simulink model "Copy_of_modelo_completo"  (R2021a)
settings: Solver=VariableStepAuto  StartTime=0.0  StopTime=10.0  RelTol=1e-3
values from neighbouring files (symbols this model uses):
  bah = Meqh*nh*w_posh    (= 720000)    [Data.m]
  bat = Meqt*nt*w_post    (= 675000)    [Data.m]
  bcx = 1000.0    (= 1000)    [Data.m]
  bcy = 500.0    (= 500)    [Data.m]
  beqh = 18.0    (= 18)    [Data.m]
  beqhd = bh + ((beqh*(rth^2))/(Rd^2))    (= 28800)    [Data.m]
  beqt = bt + (beq_rot*rt^2)/(Rw^2)    (= 27000)    [Data.m]
  bw = 30000.0    (= 30000)    [Data.m]
  cont_mass = max_m    (= 50000)    [Data.m]
  ddxmax = 1    [Data.m]
  ddxmin = -1    [Data.m]
  g = 9.80665    [Data.m]    (also in PD_balanceo.m = 9.81)
  Kcy = 1.3e6    (= 1300000)    [Data.m]
  Ksah = Meqh*nh*w_posh^2    (= 4318720.37915)    [Data.m]
  Ksat = Meqt*nt*w_post^2    (= 3088564.26247)    [Data.m]
  Ksiah = Meqh*w_posh^3    (= 10361858.7296)    [Data.m]
  Ksiat = Meqt*w_post^3    (= 5652876.56499)    [Data.m]
  Kw = 1800000.0    (= 1800000)    [Data.m]
  Meqh = Mh + (Jmh*rth^2 + Jd)/Rd^2    (= 48014.2222222)    [Data.m]
  Meqt = mt + (Jw+Jm*rt^2)/(Rw^2)    (= 59008)    [Data.m]
  Rd = 0.75    [Data.m]
  rt = 15.0    (= 15)    [Data.m]    (also in main.m = 0)
  rth = 30.0    (= 30)    [Data.m]
  Rw = 0.5    [Data.m]    (also in main.m = 0)
  sp_mass = 15000.0    (= 15000)    [Data.m]
  yt0 = 45.0    (= 45)    [Data.m]
settings Model: Creator=Mariano  LastModifiedBy=facu_

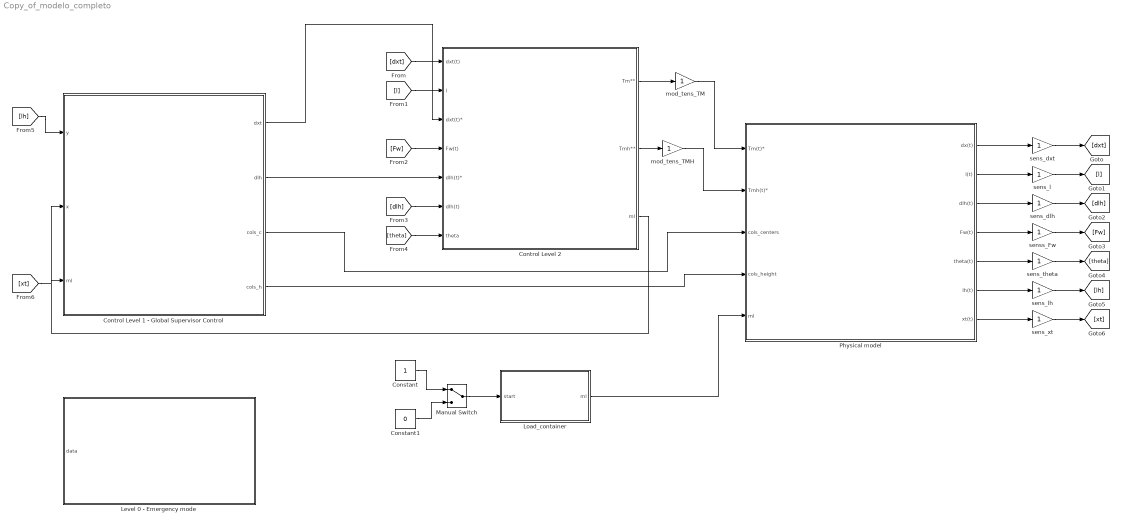
== system Copy_of_modelo_completo ==
  Constant : Constant
  Constant1 : Constant  Value=0
  Control Level 1 - Global Supervisor Control : Stateflow chart  TreatAsAtomicUnit=on
  Control Level 2 : Subsystem
  Level 0 - Emergency mode : Stateflow chart  TreatAsAtomicUnit=on
  Load_container : Subsystem
  Manual Switch : ManualSwitch
  Physical model : Subsystem
  mod_tens_TM : Gain
  mod_tens_TMH : Gain
  sens_dlh : Gain
  sens_dxt : Gain
  sens_l : Gain
  sens_lh : Gain
  sens_theta : Gain
  sens_xt : Gain
  senss_Fw : Gain
  wires:
  Control Level 2/1(Tm**) -> mod_tens_TM/1
  Control Level 2/2(Tmh**) -> mod_tens_TMH/1
  Control Level 1 - Global Supervisor Control/1(dxt) -> Control Level 2/3(dxt(t)*)
  Control Level 1 - Global Supervisor Control/2(dlh) -> Control Level 2/5(dlh(t)*)
  Physical model/1(dx(t)) -> sens_dxt/1
  Physical model/2(l(t)) -> sens_l/1
  Physical model/3(dlh(t)) -> sens_dlh/1
  Physical model/4(Fw(t)) -> senss_Fw/1
  Physical model/5(theta(t)) -> sens_theta/1
  [dxt] -> Control Level 2/1(dxt(t))
  [l] -> Control Level 2/2(l)
  [Fw] -> Control Level 2/4(Fw(t))
  [dlh] -> Control Level 2/6(dlh(t))
  [theta] -> Control Level 2/7(theta)
  Physical model/6(lh(t)) -> sens_lh/1
  Physical model/7(xt(t)) -> sens_xt/1
  [lh] -> Control Level 1 - Global Supervisor Control/1(y)
  [xt] -> Control Level 1 - Global Supervisor Control/2(x)
  sens_dxt/1 -> [dxt]
  sens_l/1 -> [l]
  sens_dlh/1 -> [dlh]
  senss_Fw/1 -> [Fw]
  sens_theta/1 -> [theta]
  sens_lh/1 -> [lh]
  sens_xt/1 -> [xt]
  mod_tens_TM/1 -> Physical model/1(Tm(t)*)
  mod_tens_TMH/1 -> Physical model/2(Tmh(t)*)
  Control Level 1 - Global Supervisor Control/3(cols_c) -> Physical model/3(cols_centers)
  Control Level 1 - Global Supervisor Control/4(cols_h) -> Physical model/4(cols_height)
  Load_container/1(ml) -> Physical model/5(ml)
  Manual Switch/1 -> Load_container/1(start)
  Constant/1 -> Manual Switch/1
  Constant1/1 -> Manual Switch/2
  Control Level 2/3(ml) -> Control Level 1 - Global Supervisor Control/3(ml)

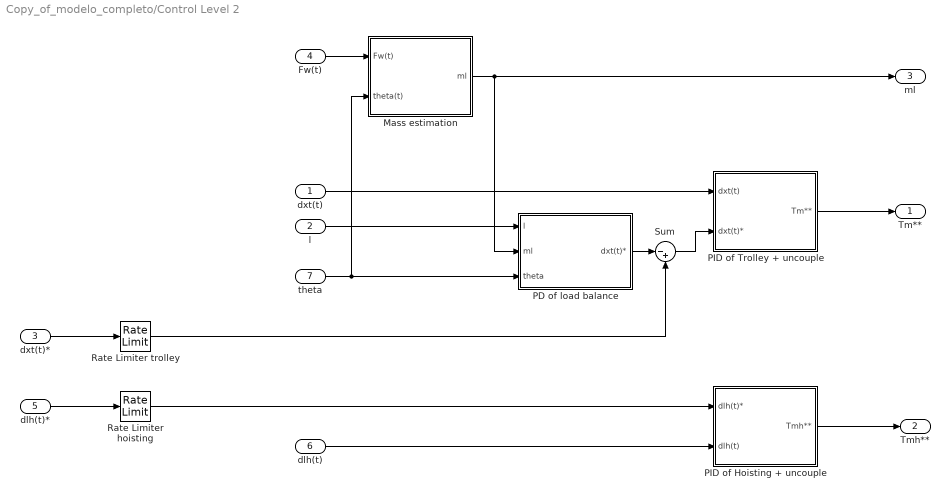
== system Copy_of_modelo_completo/Control Level 2 ==
  dxt(t) : Inport
  l : Inport  Port=2
  dxt(t)* : Inport  Port=3
  Fw(t) : Inport  Port=4
  dlh(t)* : Inport  Port=5
  dlh(t) : Inport  Port=6
  theta : Inport  Port=7
  Mass estimation : Subsystem
  "PD of load balance " : Subsystem
  "PID of Hoisting + uncouple " : Subsystem
  "PID of Trolley + uncouple " : Subsystem
  Rate Limiter hoisting : RateLimiter  RisingSlewLimit=ddxmax  FallingSlewLimit=ddxmin
  Rate Limiter trolley : RateLimiter  RisingSlewLimit=ddxmax  FallingSlewLimit=ddxmin
  Sum : Sum  Inputs=|-+
  Tm** : Outport
  Tmh** : Outport  Port=2
  ml : Outport  Port=3
  wires:
  dlh(t)*/1 -> Rate Limiter hoisting/1
  Fw(t)/1 -> Mass estimation/1(Fw(t))
  "PID of Trolley + uncouple "/1(Tm**) -> Tm**/1
  Mass estimation/1(ml) -> ml/1, "PD of load balance "/2(ml)
  "PD of load balance "/1(dxt(t)*) -> Sum/1
  Sum/1 -> "PID of Trolley + uncouple "/2(dxt(t)*)
  dxt(t)/1 -> "PID of Trolley + uncouple "/1(dxt(t))
  "PID of Hoisting + uncouple "/1(Tmh**) -> Tmh**/1
  dxt(t)*/1 -> Rate Limiter trolley/1
  l/1 -> "PD of load balance "/1(l)
  theta/1 -> Mass estimation/2(theta(t)), "PD of load balance "/3(theta)
  Rate Limiter trolley/1 -> Sum/2
  Rate Limiter hoisting/1 -> "PID of Hoisting + uncouple "/1(dlh(t)*)
  dlh(t)/1 -> "PID of Hoisting + uncouple "/2(dlh(t))

== system Copy_of_modelo_completo/Load_container ==
  start : Inport
  Sum : Sum  Inputs=|++
  Switch : Switch  Criteria=u2 > Threshold
  no_container : Constant  Value=0
  random_container_mass : Constant  Value=cont_mass
  spreader mass : Constant  Value=sp_mass
  ml : Outport
  wires:
  no_container/1 -> Switch/1
  spreader mass/1 -> Sum/2
  random_container_mass/1 -> Switch/3
  Switch/1 -> Sum/1
  Sum/1 -> ml/1
  start/1 -> Switch/2

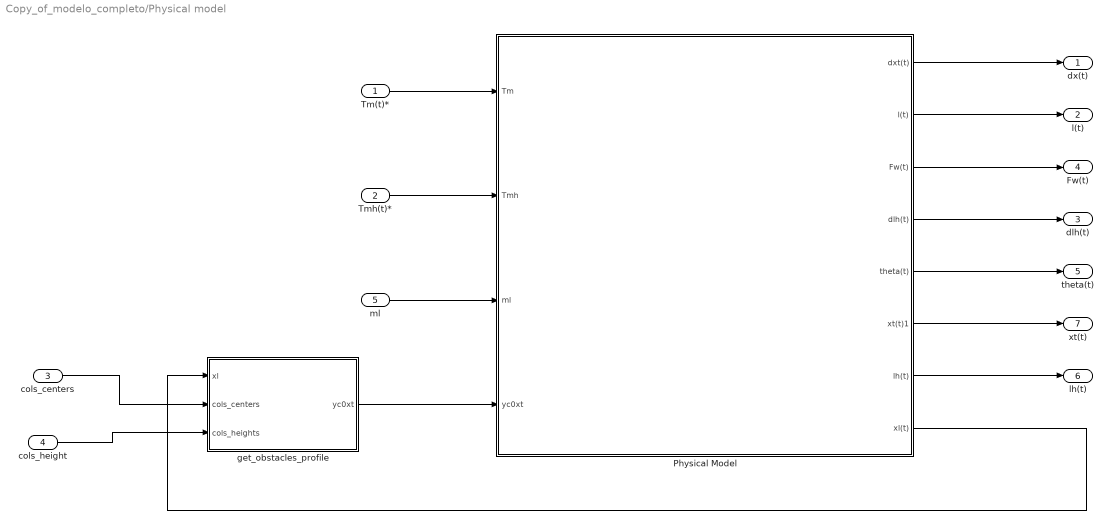
== system Copy_of_modelo_completo/Physical model ==
  Tm(t)* : Inport
  Tmh(t)* : Inport  Port=2
  cols_centers : Inport  Port=3
  cols_height : Inport  Port=4
  ml : Inport  Port=5
  Physical Model : Subsystem
  get_obstacles_profile : MATLAB Function  TreatAsAtomicUnit=on
  dx(t) : Outport
  l(t) : Outport  Port=2
  dlh(t) : Outport  Port=3
  Fw(t) : Outport  Port=4
  theta(t) : Outport  Port=5
  lh(t) : Outport  Port=6
  xt(t) : Outport  Port=7
  wires:
  Physical Model/4(dlh(t)) -> dlh(t)/1
  Physical Model/2(l(t)) -> l(t)/1
  Physical Model/1(dxt(t)) -> dx(t)/1
  Physical Model/3(Fw(t)) -> Fw(t)/1
  Physical Model/5(theta(t)) -> theta(t)/1
  Physical Model/6(xt(t)1) -> xt(t)/1
  Physical Model/7(lh(t)) -> lh(t)/1
  Tmh(t)*/1 -> Physical Model/2(Tmh)
  Tm(t)*/1 -> Physical Model/1(Tm)
  ml/1 -> Physical Model/3(ml)
  get_obstacles_profile/1(yc0xt) -> Physical Model/4(yc0xt)
  Physical Model/8(xl(t)) -> get_obstacles_profile/1(xl)
  cols_centers/1 -> get_obstacles_profile/2(cols_centers)
  cols_height/1 -> get_obstacles_profile/3(cols_heights)

== system Copy_of_modelo_completo/Control Level 2/Mass estimation ==
  Fw(t) : Inport
  theta(t) : Inport  Port=2
  Constant : Constant  Value=g
  Divide : Product  Inputs=*/
  Product : Product
  Trigonometric Function : Trigonometry
  ml : Outport
  wires:
  theta(t)/1 -> Trigonometric Function/1
  Trigonometric Function/1 -> Product/2
  Fw(t)/1 -> Product/1
  Divide/1 -> ml/1
  Product/1 -> Divide/1
  Constant/1 -> Divide/2

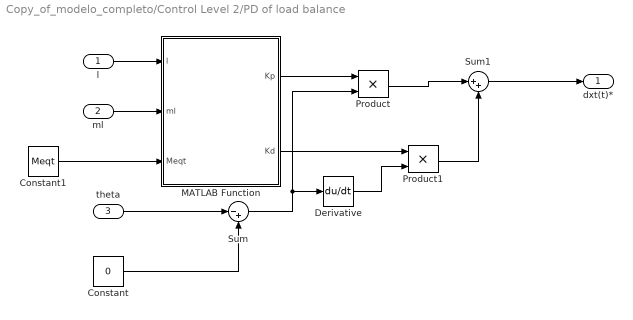
== system Copy_of_modelo_completo/Control Level 2/PD of load balance  ==
  l : Inport
  ml : Inport  Port=2
  theta : Inport  Port=3
  Constant : Constant  Value=0
  Constant1 : Constant  Value=Meqt
  Derivative : Derivative
  MATLAB Function : MATLAB Function  TreatAsAtomicUnit=on
  Product : Product
  Product1 : Product
  Sum : Sum  Inputs=|-+
  Sum1 : Sum  Inputs=|++
  dxt(t)* : Outport
  wires:
  theta/1 -> Sum/1
  Constant/1 -> Sum/2
  ml/1 -> MATLAB Function/2(ml)
  Sum/1 -> Product/2, Derivative/1
  Product1/1 -> Sum1/2
  Product/1 -> Sum1/1
  Sum1/1 -> dxt(t)*/1
  MATLAB Function/2(Kd) -> Product1/1
  MATLAB Function/1(Kp) -> Product/1
  Derivative/1 -> Product1/2
  l/1 -> MATLAB Function/1(l)
  Constant1/1 -> MATLAB Function/3(Meqt)

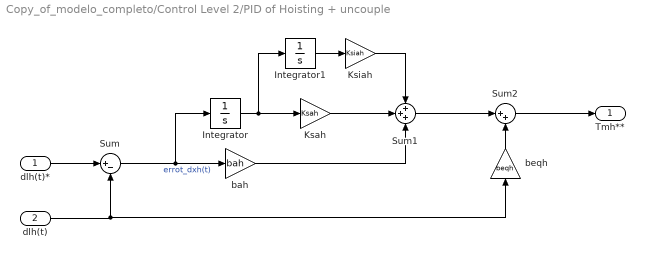
== system Copy_of_modelo_completo/Control Level 2/PID of Hoisting + uncouple  ==
  dlh(t)* : Inport
  dlh(t) : Inport  Port=2
  Integrator : Integrator
  Integrator1 : Integrator
  Ksah : Gain  Gain=Ksah
  Ksiah : Gain  Gain=Ksiah
  Sum : Sum  Inputs=|+-
  Sum1 : Sum  Inputs=+++
  Sum2 : Sum  Inputs=|++
  bah : Gain  Gain=bah
  beqh : Gain  Gain=beqh
  Tmh** : Outport
  wires:
  Sum/1 -> bah/1, Integrator/1  "errot_dxh(t)"
  dlh(t)*/1 -> Sum/1
  Sum1/1 -> Sum2/1
  dlh(t)/1 -> beqh/1, Sum/2
  Integrator/1 -> Integrator1/1, Ksah/1
  bah/1 -> Sum1/3
  Ksah/1 -> Sum1/2
  Integrator1/1 -> Ksiah/1
  Ksiah/1 -> Sum1/1
  beqh/1 -> Sum2/2
  Sum2/1 -> Tmh**/1

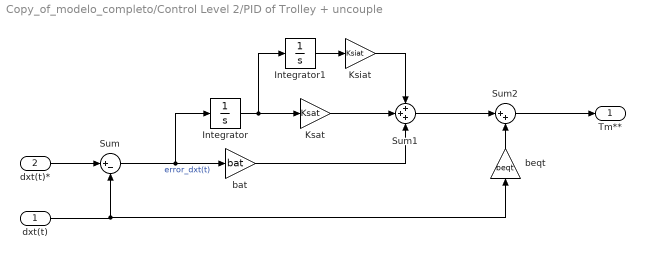
== system Copy_of_modelo_completo/Control Level 2/PID of Trolley + uncouple  ==
  dxt(t) : Inport
  dxt(t)* : Inport  Port=2
  Integrator : Integrator
  Integrator1 : Integrator
  Ksat : Gain  Gain=Ksat
  Ksiat : Gain  Gain=Ksiat
  Sum : Sum  Inputs=|+-
  Sum1 : Sum  Inputs=+++
  Sum2 : Sum  Inputs=|++
  bat : Gain  Gain=bat
  beqt : Gain  Gain=beqt
  Tm** : Outport
  wires:
  Sum/1 -> bat/1, Integrator/1  "error_dxt(t)"
  dxt(t)*/1 -> Sum/1
  Sum1/1 -> Sum2/1
  dxt(t)/1 -> beqt/1, Sum/2
  Integrator/1 -> Integrator1/1, Ksat/1
  bat/1 -> Sum1/3
  Ksat/1 -> Sum1/2
  Integrator1/1 -> Ksiat/1
  Ksiat/1 -> Sum1/1
  beqt/1 -> Sum2/2
  Sum2/1 -> Tm**/1

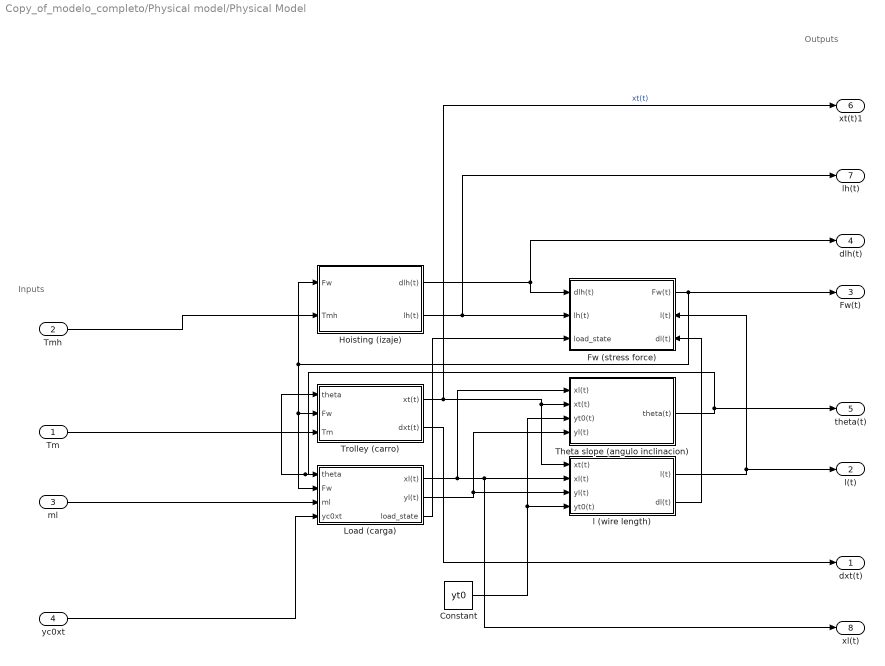
== system Copy_of_modelo_completo/Physical model/Physical Model ==
  note: Inputs
  note: Outputs
  Tm : Inport
  Tmh : Inport  Port=2
  ml : Inport  Port=3
  yc0xt : Inport  Port=4
  Constant : Constant  Value=yt0
  Fw (stress force) : Subsystem
      settings: PortSchema="{\"entries\":[{\"content\":{\"sides\":[{\"content\":{\"connectorIds\":[\"In1\",\"In2\",\"In3\"]},\"type\":\"ConnectorPlacement.EquallySpacedRectSide\",\"uuid\":\"ba23d8a5-df88-4a98-9228-1a95ef0572d6\"},{\"content\":{\"connectorIds\":[\"Out1\",\"In4\",\"In5\"],\"side\":\"RIGHT\"},\"type\":\"ConnectorPlacement.EquallySpacedRectSide\",\"uuid\":\"c1b2cc2a-1d19-40da-89ec-405abbf25b58\"},{\"content\":{\"connectorIds\":[],\"side\":\"TOP\"},\"type\":\"ConnectorPlacement.EquallySpacedRectSide\",\"uuid\":\"8c283652-7118-429a-8320-3bc0966db205\"}]},\"type\":\"ConnectorPlacement.EquallySpacedConnector\",\"uuid\":\"7ebc4a5f-6f80-4333-9ee6-9a21b2f2a5d0\"}],\"packageUris\":[\"http://schema.mathworks.com/mf0/Connector/R2020b\"],\"version\":\"1.0\"}"
  Hoisting (izaje) : Subsystem
  Load (carga) : Subsystem
  Theta slope (angulo inclinacion) : Subsystem
  Trolley (carro) : Subsystem
  l (wire length) : Subsystem
  dxt(t) : Outport
  l(t) : Outport  Port=2
  Fw(t) : Outport  Port=3
  dlh(t) : Outport  Port=4
  theta(t) : Outport  Port=5
  xt(t)1 : Outport  Port=6
  lh(t) : Outport  Port=7
  xl(t) : Outport  Port=8
  wires:
  Theta slope (angulo inclinacion)/1(theta(t)) -> theta(t)/1, Trolley (carro)/1(theta), Load (carga)/1(theta)
  Load (carga)/1(xl(t)) -> xl(t)/1, l (wire length)/2(xl(t)), Theta slope (angulo inclinacion)/1(xl(t))
  Hoisting (izaje)/2(lh(t)) -> lh(t)/1, Fw (stress force)/2(lh(t))
  Trolley (carro)/1(xt(t)) -> xt(t)1/1, l (wire length)/1(xt(t)), Theta slope (angulo inclinacion)/2(xt(t))  "xt(t)"
  Fw (stress force)/1(Fw(t)) -> Trolley (carro)/2(Fw), Load (carga)/2(Fw), Hoisting (izaje)/1(Fw), Fw(t)/1
  Constant/1 -> Theta slope (angulo inclinacion)/3(yt0(t)), l (wire length)/4(yt0(t))
  Load (carga)/2(yl(t)) -> Theta slope (angulo inclinacion)/4(yl(t)), l (wire length)/3(yl(t))
  l (wire length)/1(l(t)) -> l(t)/1, Fw (stress force)/4(l(t))
  ml/1 -> Load (carga)/3(ml)
  l (wire length)/2(dl(t)) -> Fw (stress force)/5(dl(t))
  Tmh/1 -> Hoisting (izaje)/2(Tmh)
  Tm/1 -> Trolley (carro)/3(Tm)
  Hoisting (izaje)/1(dlh(t)) -> Fw (stress force)/1(dlh(t)), dlh(t)/1
  Trolley (carro)/2(dxt(t)) -> dxt(t)/1
  Load (carga)/3(load_state) -> Fw (stress force)/3(load_state)
  yc0xt/1 -> Load (carga)/4(yc0xt)

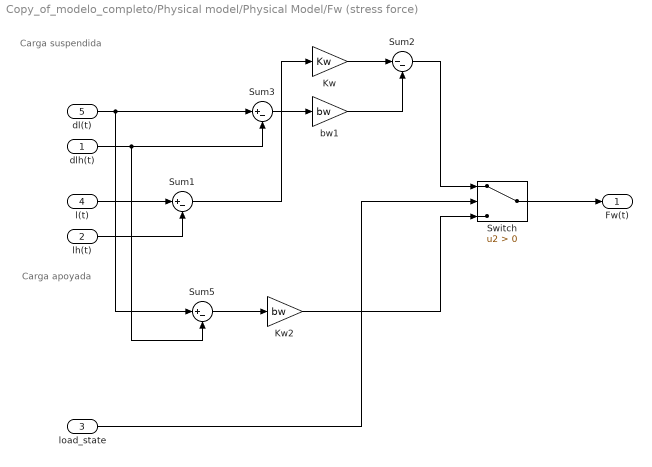
== system Copy_of_modelo_completo/Physical model/Physical Model/Fw (stress force) ==
  note: Carga suspendida
  note: Carga apoyada
  dlh(t) : Inport
  lh(t) : Inport  Port=2
  load_state : Inport  Port=3
  l(t) : Inport  Port=4
  dl(t) : Inport  Port=5
  Kw : Gain  Gain=Kw
  Kw2 : Gain  Gain=bw
  Sum1 : Sum  Inputs=|+-
  Sum2 : Sum  Inputs=|--
  Sum3 : Sum  Inputs=|+-
  Sum5 : Sum  Inputs=|+-
  Switch : Switch  Criteria=u2 > Threshold
  bw1 : Gain  Gain=bw
  Fw(t) : Outport
  wires:
  Switch/1 -> Fw(t)/1
  l(t)/1 -> Sum1/1
  lh(t)/1 -> Sum1/2
  Sum1/1 -> Kw/1
  Sum3/1 -> bw1/1
  bw1/1 -> Sum2/2
  Kw/1 -> Sum2/1
  Sum2/1 -> Switch/1
  Sum5/1 -> Kw2/1
  dlh(t)/1 -> Sum5/2, Sum3/2
  dl(t)/1 -> Sum5/1, Sum3/1
  Kw2/1 -> Switch/3
  load_state/1 -> Switch/2

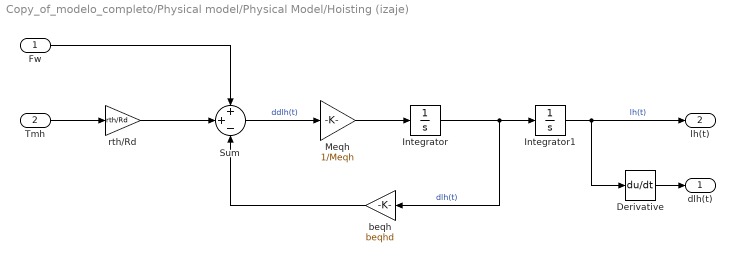
== system Copy_of_modelo_completo/Physical model/Physical Model/Hoisting (izaje) ==
  Fw : Inport
  Tmh : Inport  Port=2
  Derivative : Derivative
  Integrator : Integrator
  Integrator1 : Integrator
  Meqh : Gain  Gain=1/Meqh
  Sum : Sum  Inputs=++-
  beqh : Gain  Gain=beqhd
  rth/Rd : Gain  Gain=rth/Rd
  dlh(t) : Outport
  lh(t) : Outport  Port=2
  wires:
  Fw/1 -> Sum/1
  Tmh/1 -> rth/Rd/1
  rth/Rd/1 -> Sum/2
  Sum/1 -> Meqh/1  "ddlh(t)"
  Meqh/1 -> Integrator/1
  Integrator/1 -> beqh/1, Integrator1/1  "dlh(t)"
  Integrator1/1 -> Derivative/1, lh(t)/1  "lh(t)"
  beqh/1 -> Sum/3
  Derivative/1 -> dlh(t)/1

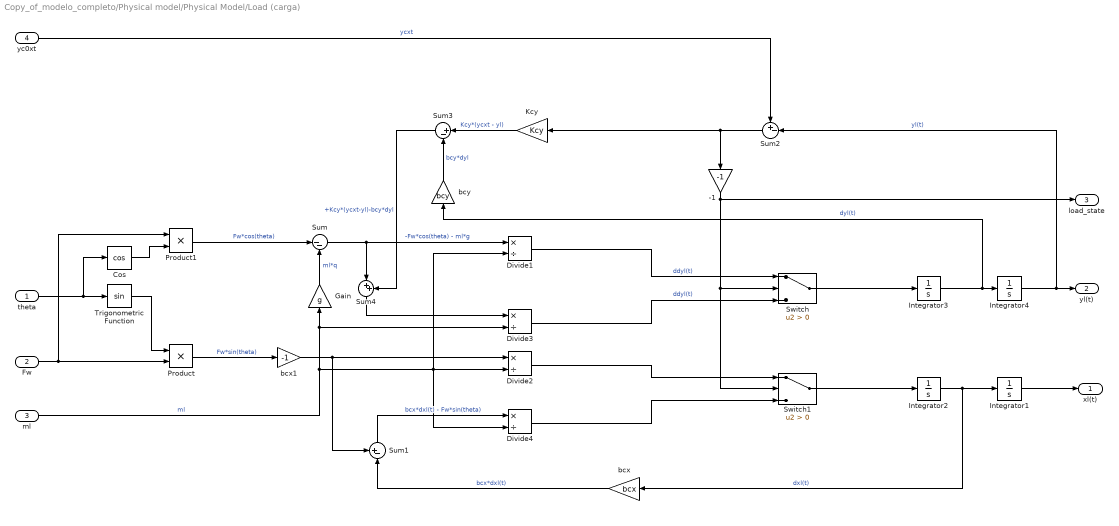
== system Copy_of_modelo_completo/Physical model/Physical Model/Load (carga) ==
  theta : Inport
  Fw : Inport  Port=2
  ml : Inport  Port=3
  yc0xt : Inport  Port=4
  -1 : Gain  Gain=-1
  Cos : Trigonometry  Operator=cos
  Divide{1..4} (4 alike) : Product  Inputs=*/
  Gain : Gain  Gain=g
  Integrator{1..4} (4 alike) : Integrator
  Kcy : Gain  Gain=Kcy
  Product : Product
  Product1 : Product
  Sum : Sum  Inputs=|--
  Sum1 : Sum  Inputs=+-|
  Sum2 : Sum  Inputs=+-|
  Sum3 : Sum  Inputs=|+-
  Sum4 : Sum  Inputs=|++
  Switch : Switch  Criteria=u2 > Threshold
  Switch1 : Switch  Criteria=u2 > Threshold
  Trigonometric Function : Trigonometry
  bcx : Gain  Gain=bcx
  bcx1 : Gain  Gain=-1
  bcy : Gain  Gain=bcy
  xl(t) : Outport
  yl(t) : Outport  Port=2
  load_state : Outport  Port=3
  wires:
  theta/1 -> Trigonometric Function/1, Cos/1
  Trigonometric Function/1 -> Product/1
  Fw/1 -> Product/2, Product1/1
  Integrator1/1 -> xl(t)/1
  Integrator2/1 -> bcx/1, Integrator1/1  "dxl(t)"
  ml/1 -> Divide4/2, Divide2/2, Divide1/2, Divide3/2, Gain/1  "ml"
  Product/1 -> bcx1/1  "Fw*sin(theta)"
  Cos/1 -> Product1/2
  Product1/1 -> Sum/1  "Fw*cos(theta)"
  Sum/1 -> Sum4/1, Divide1/1  "-Fw*cos(theta) - ml*g"
  Integrator3/1 -> bcy/1, Integrator4/1  "dyl(t)"
  Integrator4/1 -> Sum2/2, yl(t)/1  "yl(t)"
  Gain/1 -> Sum/2  "ml*q"
  Divide1/1 -> Switch/1  "ddyl(t)"
  Switch/1 -> Integrator3/1
  Switch1/1 -> Integrator2/1
  Divide2/1 -> Switch1/1
  Divide4/1 -> Switch1/3
  Divide3/1 -> Switch/3  "ddyl(t)"
  bcx1/1 -> Sum1/1, Divide2/1
  bcx/1 -> Sum1/2  "bcx*dxl(t)"
  Sum1/1 -> Divide4/1  "bcx*dxl(t) - Fw*sin(theta)"
  Sum2/1 -> Kcy/1, -1/1
  yc0xt/1 -> Sum2/1  "ycxt"
  Kcy/1 -> Sum3/1  "Kcy*(ycxt - yl)"
  bcy/1 -> Sum3/2  "bcy*dyl"
  Sum4/1 -> Divide3/1
  Sum3/1 -> Sum4/2  "+Kcy*(ycxt-yl)-bcy*dyl"
  -1/1 -> load_state/1, Switch1/2, Switch/2

== system Copy_of_modelo_completo/Physical model/Physical Model/Theta slope (angulo inclinacion) ==
  xl(t) : Inport
  xt(t) : Inport  Port=2
  yt0(t) : Inport  Port=3
  yl(t) : Inport  Port=4
  Atan2 : Trigonometry  Operator=atan2
  Sum : Sum  Inputs=-+
  Sum1 : Sum  Inputs=+-
  theta(t) : Outport
  wires:
  yt0(t)/1 -> Sum/1
  yl(t)/1 -> Sum/2
  xl(t)/1 -> Sum1/1
  xt(t)/1 -> Sum1/2
  Sum1/1 -> Atan2/1  "xl-xt"
  Sum/1 -> Atan2/2  "yl-yt"
  Atan2/1 -> theta(t)/1

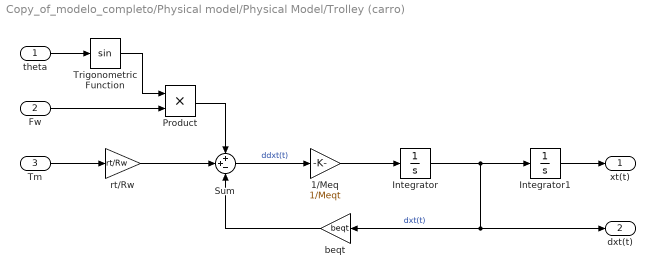
== system Copy_of_modelo_completo/Physical model/Physical Model/Trolley (carro) ==
  theta : Inport
  Fw : Inport  Port=2
  Tm : Inport  Port=3
  1/Meq : Gain  Gain=1/Meqt
  Integrator : Integrator
  Integrator1 : Integrator
  Product : Product
  Sum : Sum  Inputs=++-
  Trigonometric Function : Trigonometry
  beqt : Gain  Gain=beqt
  rt/Rw : Gain  Gain=rt/Rw
  xt(t) : Outport
  dxt(t) : Outport  Port=2
  wires:
  theta/1 -> Trigonometric Function/1
  Trigonometric Function/1 -> Product/1
  Fw/1 -> Product/2
  Product/1 -> Sum/1
  Tm/1 -> rt/Rw/1
  rt/Rw/1 -> Sum/2
  Sum/1 -> 1/Meq/1  "ddxt(t)"
  1/Meq/1 -> Integrator/1
  Integrator/1 -> Integrator1/1, dxt(t)/1, beqt/1  "dxt(t)"
  Integrator1/1 -> xt(t)/1
  beqt/1 -> Sum/3

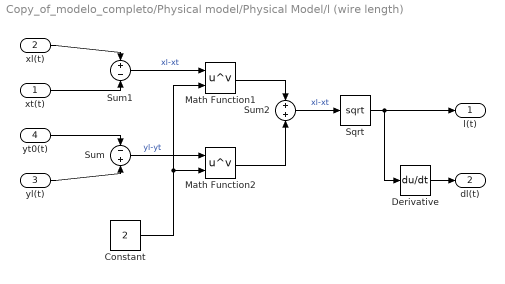
== system Copy_of_modelo_completo/Physical model/Physical Model/l (wire length) ==
  xt(t) : Inport
  xl(t) : Inport  Port=2
  yl(t) : Inport  Port=3
  yt0(t) : Inport  Port=4
  Constant : Constant  Value=2
  Derivative : Derivative
  Math Function1 : Math  Operator=pow  SignedPower=on  SaturateOnIntegerOverflow=on
  Math Function2 : Math  Operator=pow  SignedPower=on  SaturateOnIntegerOverflow=on
  Sqrt : Sqrt  SaturateOnIntegerOverflow=on
  Sum : Sum  Inputs=-+
  Sum1 : Sum  Inputs=+-
  Sum2 : Sum
  l(t) : Outport
  dl(t) : Outport  Port=2
  wires:
  yt0(t)/1 -> Sum/1
  yl(t)/1 -> Sum/2
  xl(t)/1 -> Sum1/1
  xt(t)/1 -> Sum1/2
  Sqrt/1 -> Derivative/1, l(t)/1
  Sum1/1 -> Math Function1/1  "xl-xt"
  Sum/1 -> Math Function2/1  "yl-yt"
  Math Function1/1 -> Sum2/1
  Math Function2/1 -> Sum2/2
  Sum2/1 -> Sqrt/1  "xl-xt"
  Derivative/1 -> dl(t)/1
  Constant/1 -> Math Function2/2, Math Function1/2

== stateflow chart Copy_of_modelo_completo/Level 0 - Emergency mode ==
  data: data input

== matlab function Copy_of_modelo_completo/Control Level 2/PD of load balance /MATLAB Function ==
  data: l input; Kp output; ml input; Kd output; Meqt input
function [Kp,Kd] = fcn(l, ml,Meqt)
    wn=800;
    g=9.81;
    Kd = l - ( (Meqt*g)/((wn^2)*(ml+Meqt)) ) ;
    Kp = 2*wn*1*(-l + Kd);
end

== stateflow chart Copy_of_modelo_completo/Control Level 1 - Global Supervisor Control ==
  note: Descripcion variables:
      | CARRO (TROLLEY):
      | - move_t -> (variable,int) boton para mover el carro en x.
      | - dx -> (variable,double) velocidad actual del carro (variable)
      | - VXt -> velocidad máxima del carro (es una constante, que al multiplicarla por bot_t modifica el valor de la velocidad real de carro.)
      | - limits_t -> (variable,bool) la variable cambia al valor 1 si se alcanzan los limites de movimiento del carro.
      |
      | IZAJE (HOISTING):
      | - move_h ->(variable,int) boton para izar la carga.
      | - dy -> (variable,double) velocidad actual del izaje.
      | - VYh -> (constante) velocidad máxima que puede alcanzar el izaje.
      | - limits_h -> (variable,bool) la variable cambia al valor 1 si se alcanzan los limites de movimiento del izaje.
      |
      | Descripcion de bloques:
      | - ALL_MANUAL:
      | Es el modo manual por defecto, el operario puede manejar el trolley y el hoisting con 2 botones. El boton move_t se encarga de mover el trolley y el boton move_h de izar la carga.
      | - HYRBID_MANUAL:
      | Es el modo manual que esta presente en los ciclos simple o doble. Es decir, esta intercalado con el modo automático
  note: Descripción de ciclos:
      | -SIMPLE:
      | O se carga o se descarga, es decir: Si estoy cargando el barco, en el tramo muelle -> barco llevo un contenedor, pero vuelvo vacio. Es decir que el tramo barco -> muelle es sin ningun contenedor. Lo mismo sucederia si estoy descargando el barco: el tramo barco -> muelle es con un contenedor cargado, pero el tramo muelle -> barco es en vacio.
      | - DOBLE:
      | Se puede cargar y descargar en el mismo ciclo de trabajo. Es decir, que el tramo muelle -> barco es con un contenedor cargado, y el tramo barco -> muelle también. Por ende, se permite una carga intermedia antes de volver al muelle.
      |
      | ETAPAS DE LA TRAYECTORIA:
      | Cada stage se va aactivando dependiendo del punto de la trayectoria en el que se encuentra el barco
      | - STAGE 1 -> ground - el contenedor esta en tierra
      | - STAGE 2 -> el contenedor se encuentra en el aire (sobre muelle), en el punto de transicion manual a automatico.
      | - STAGE 3 -> el contenedor se enceuntra en el aire (sobre barco) ,en el punto de transicion automatico a manual.
      | - STAGE 4 -> el contenedor se encuentra en el barco.
  state LEVEL1
    state MOVEMENT [parallel]
      settings: executionOrder=1
      state HYBRID_MANUAL
        state HOISTING [parallel]
          entry: limits_h=0;
          settings: executionOrder=1
          state MOVE
            during:
            dlh=1.5;
          state STOP
            entry:
            dlh=0;
          (default) -> LEVEL1.MOVEMENT.HYBRID_MANUAL.HOISTING.MOVE
          LEVEL1.MOVEMENT.HYBRID_MANUAL.HOISTING.STOP -> LEVEL1.MOVEMENT.HYBRID_MANUAL.HOISTING.MOVE : [limits_h==0]
          LEVEL1.MOVEMENT.HYBRID_MANUAL.HOISTING.MOVE -> LEVEL1.MOVEMENT.HYBRID_MANUAL.HOISTING.STOP : [limits_h==1]
        state TROLLEY [parallel]
          entry: limits_t=0;
          settings: executionOrder=2
          state STOP
            entry:
            dxt=0;
          state MOVE
            during:
            dxt=4;
          (default) -> LEVEL1.MOVEMENT.HYBRID_MANUAL.TROLLEY.MOVE
          LEVEL1.MOVEMENT.HYBRID_MANUAL.TROLLEY.STOP -> LEVEL1.MOVEMENT.HYBRID_MANUAL.TROLLEY.MOVE : [limits_t==0]
          LEVEL1.MOVEMENT.HYBRID_MANUAL.TROLLEY.MOVE -> LEVEL1.MOVEMENT.HYBRID_MANUAL.TROLLEY.STOP : [limits_t==1]
      (default) -> HYBRID_MANUAL
  (default) -> LEVEL1
  data: dxt output size=1; dlh output size=1; y input; x input; cols_c output size=1; cols_h output size=1; cols_centers local; charge local; cols_height local; double_cycle local; p0 local; p1 local; p2 local; p3 local; p4 local; p5 local; p6 local; p7 local; single_cycle local; current_stage local; limits_h local; limits_t local; prev_stage local; VH_MAX local; VT_MAX local; ml input

== matlab function Copy_of_modelo_completo/Physical model/get_obstacles_profile ==
  data: xl input; yc0xt output; cols_centers input; cols_heights input
function yc0xt = get_obstacles_profile(xl, cols_centers, cols_heights)

%{
@type MATLAB function called from SIMULINK
@name get_obstacles_profile
@description - Obtiene el perfil de obstaculos 
@params {float,simulation} xl - valor en tiempo real de la posocion del
carro
@params {array} cols_centers - Contiene las coordenadas de los centros de
cada columna. Array de 1xN , con N = cantidad de columnas
@params {cols_heights} - Altura de cada columna respecto del punto 0,0.
@returns {float} yc0xt - Valor en altura del obstaculo para la coordenada
xl, en el instante de tiempo t actual.
%}


if (xl <= 0) % Si estamos sobre el muelle no hay obstaculos, entonces ycxt=0
    yc0xt = 0;

elseif (xl > 0) % Si estamos por encima del barco
    
    
end % end ifelse

end %end function
